simulink model "pneumatic_reference"  (R2025a)
settings: Solver=ode45  StartTime=0.0  StopTime=5  MaxStep=0.002  RelTol=1e-7  AbsTol=1e-12
undefined symbols (not defined in the file): pneumatic_initial, pneumatic_parameters
settings Model: Creator=dewar  LastModifiedBy=dewar

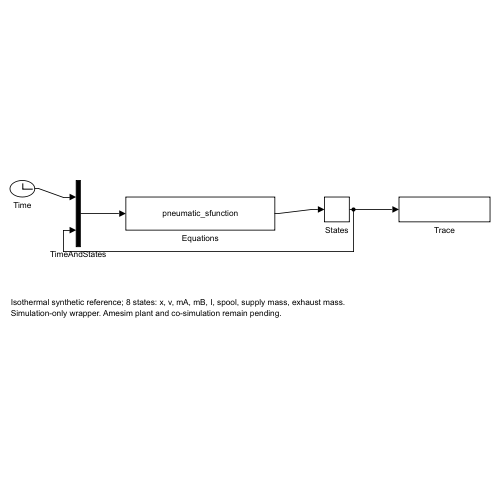
[thumbnail: Simulink's stored preview of the top-level diagram]
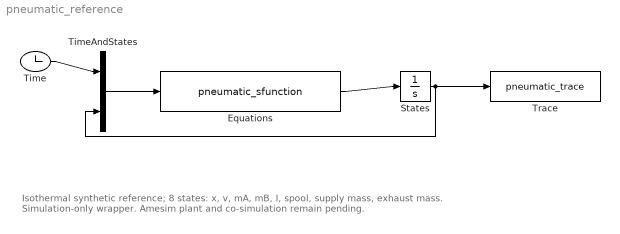
== system pneumatic_reference ==
  note: Isothermal synthetic reference; 8 states: x, v, mA, mB, I, spool, supply mass, exhaust mass.
      | Simulation-only wrapper. Amesim plant and co-simulation remain pending.
  Equations : M-S-Function  FunctionName=pneumatic_sfunction
  States : Integrator  InitialCondition=pneumatic_initial(pneumatic_parameters('tuned'))
  Time : Clock
  TimeAndStates : Mux  Inputs=2
  Trace : ToWorkspace  VariableName=pneumatic_trace  SaveFormat=Structure With Time  SampleTime=-1
  wires:
  Time/1 -> TimeAndStates/1
  States/1 -> TimeAndStates/2, Trace/1
  TimeAndStates/1 -> Equations/1
  Equations/1 -> States/1
